simulink model "lab3_test_android"  (R2019b)
settings: Solver=FixedStepAuto  StartTime=0.0  StopTime=60  RelTol=1e-3
libraries: androidsensorlib x5
settings Model: SimulationMode=external  Creator=horia  LastModifiedBy=horia
settings OptimizationCC: EnhancedBackFolding=on  PassReuseOutputArgsAs=Individual arguments  ZeroExternalMemoryAtStartup=off  ZeroInternalMemoryAtStartup=off  MaxStackSize=64  OptimizeBlockOrder=speed  DifferentSizesBufferReuse=on  OptimizationCustomize=off  EfficientTunableParamExpr=on
settings DebuggingCC: ParameterTunabilityLossMsg=error
settings HardwareCC: ProdBitPerPointer=32  ProdBitPerSizeT=32  ProdBitPerPtrDiffT=32  ProdLargestAtomicInteger=Long  ProdLargestAtomicFloat=Double  ProdWordSize=32  ProdHWDeviceType=ARM Compatible->ARM Cortex  UseEmbeddedCoderFeatures=off  UseSimulinkCoderFeatures=off
settings SFSimCC: MATLABDynamicMemAlloc=off
settings RTWCC: SystemTargetFile=ert.tlc  HardwareBoard=Android Device  TLCOptions="-aInlineSetEventsForThisBaseRateFcn=TLC_FALSE -aSuppressMultiTaskScheduler=TLC_FALSE  -aRateBasedStepFcn=0"  TemplateMakefile=ert_default_tmf  GenerateReport=on  RTWVerbose=off  Toolchain=Android SDK/NDK Tools  IncludeHyperlinkInReport=on  LaunchReport=on  GenerateTraceInfo=on  GenerateTraceReport=on  GenerateTraceReportSl=on  GenerateTraceReportSf=on  GenerateTraceReportEml=on
settings CodeAppCC: ForceParamTrailComments=on  IgnoreCustomStorageClasses=off  OperatorAnnotations=on  SimulinkDataObjDesc=on  SFDataObjDesc=on  InsertBlockDesc=on
settings ERTTargetCC: SupportNonInlinedSFcns=on

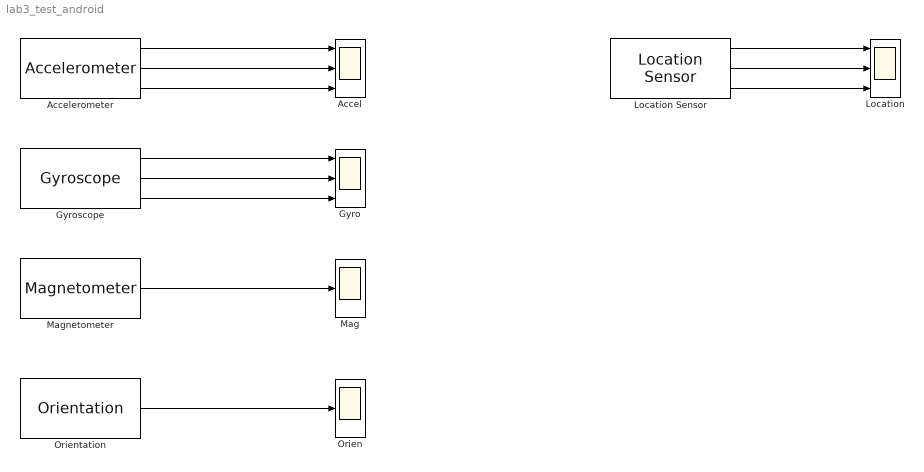
== system lab3_test_android ==
  Accel : Scope  NumInputPorts=3
  Accelerometer : androidsensorlib/Accelerometer  OutputVector=off  SampleTime=0.1  BlockPlatform=Android
      settings: SourceProductName=Simulink Support Package for Android Devices  SourceProductBaseCode=ANDROID
  Gyro : Scope  NumInputPorts=3
  Gyroscope : androidsensorlib/Gyroscope  OutputVector=off  SampleTime=0.1  BlockPlatform=Android
      settings: SourceProductName=Simulink Support Package for Android Devices  SourceProductBaseCode=ANDROID
  Location : Scope  NumInputPorts=3
  Location Sensor : androidsensorlib/Location Sensor  OutputVector=off  SampleTime=0.1  BlockPlatform=Android
      settings: SourceProductName=Simulink Support Package for Android Devices  SourceProductBaseCode=ANDROID
  Mag : Scope
  Magnetometer : androidsensorlib/Magnetometer  SampleTime=0.1  SimulateUsing=Code generation
      settings: SourceProductName=Simulink Support Package for Android Devices  SourceProductBaseCode=ANDROID
  Orien : Scope
  Orientation : androidsensorlib/Orientation  SampleTime=0.1  SimulateUsing=Code generation
      settings: SourceProductName=Simulink Support Package for Android Devices  SourceProductBaseCode=ANDROID
  wires:
  Accelerometer/1 -> Accel/1
  Accelerometer/2 -> Accel/2
  Accelerometer/3 -> Accel/3
  Gyroscope/1 -> Gyro/1
  Gyroscope/2 -> Gyro/2
  Gyroscope/3 -> Gyro/3
  Magnetometer/1 -> Mag/1
  Orientation/1 -> Orien/1
  Location Sensor/1 -> Location/1
  Location Sensor/2 -> Location/2
  Location Sensor/3 -> Location/3
